simulink model "modelo_1"  (R2023a)
settings: Solver=ode45  StartTime=0.0  StopTime=100  RelTol=1e-3
InitFcn:
  | clc;clear;close all;
  | parametros;
  | FC_detectores;
  | gen_suelo;
  | gain_CL;
values from neighbouring files (symbols this model uses):
  b_cx = 1e6    (= 1000000)    [parametros.m]
  b_cy = 1e7    (= 10000000)    [parametros.m]
  b_ha = (n_h*w_des_h+2*dseta_h*w_des_h)*(J_hEq)-b_hEq    [gain_CL.m]
  b_hb = 1e8    (= 100000000)    [parametros.m]
  b_hd = 8    [parametros.m]
  b_hEb = 2.2e9    (= 2200000000)    [parametros.m]
  b_hm = 18    [parametros.m]
  b_t = 90    [parametros.m]
  b_ta = (n_t*w_des_t+2*dseta_t*w_des_t)*(J_tEq)-b_tEq    [gain_CL.m]
  b_tb = 5e6    (= 5000000)    [parametros.m]
  b_td = 1.8    [parametros.m]
  b_tEq = b_tm+(b_td/i_t^2)+(b_t*r_td^2/i_t^2)    (= 6.027)    [parametros.m]
  b_tm = 6    [parametros.m]
  b_tw = 3e3    (= 3000)    [parametros.m]
  b_wu = 150    [parametros.m]
  FC_e = 1    [FC_detectores.m]
  g = 9.80664    [parametros.m]
  H_c = 2.5    [parametros.m]
  i_h = 22    [parametros.m]
  i_t = 30    [parametros.m]
  J_hd_hEb = 3800    [parametros.m]
  J_hm_hb = 30    [parametros.m]
  J_td = 1200    [parametros.m]
  J_tEq = J_tm_tb+(J_td/i_t^2)+((M_t)*r_td^2/i_t^2)+m_l*r_td^2/i_t^2    (= 20.8333333333)    [parametros.m]
  J_tm_tb = 7    [parametros.m]
  K_cy = 1.8e9    (= 1800000000)    [parametros.m]
  k_hsa = (w_des_h^2+2*dseta_h*w_des_h)*(J_hEq)    [gain_CL.m]
  k_hsia = (w_des_h^3)*(J_hEq)    [gain_CL.m]
  k_tsa = (w_des_t^2+2*dseta_t*w_des_t)*(J_tEq)    [gain_CL.m]
  k_tsia = (w_des_t^3)*(J_tEq)    [gain_CL.m]
  K_tw = 4.8e5    (= 480000)    [parametros.m]
  k_wu = 2.35e8    (= 235000000)    [parametros.m]
  M_cmax = 50000    [parametros.m]
  M_cmin = 2000    [parametros.m]
  M_s = 15000    [parametros.m]
  M_t = 30000    [parametros.m]
  r_hd = 0.75    [parametros.m]
  r_td = 0.50    (= 0.5)    [parametros.m]
  res = 0.01    [gen_suelo.m]
  T_hEbMax = 1.1e6    (= 1100000)    [parametros.m]
  T_s = (b_hEq/J_hEq)/2/pi/100    (= 0.000679331161018)    [parametros.m]
  T_tbMax = 5e3    (= 5000)    [parametros.m]
  v_hMax_loaded = 1.5    [FC_detectores.m]
  v_hMax_over = 1.15    [FC_detectores.m]
  v_hMax_unloaded = 3    [FC_detectores.m]
  x_tMax = 50    [FC_detectores.m]
  x_tMin = -30    [FC_detectores.m]
  y_hMax = 40    [FC_detectores.m]
  y_hMin = -20    [FC_detectores.m]
  Y_t0 = 45    [parametros.m]
libraries: simulink x10
settings Model: Creator=Usuario  LastModifiedBy=Usuario

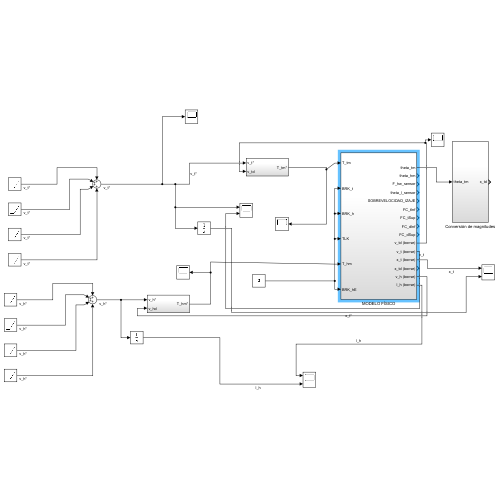
[thumbnail: Simulink's stored preview of the top-level diagram]
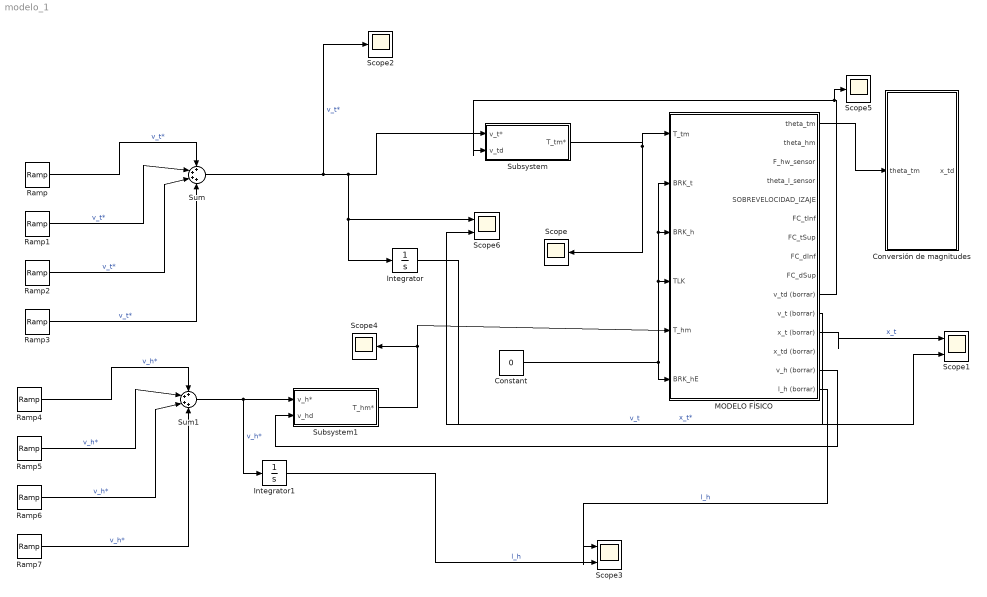
== system modelo_1 ==
  Constant : Constant  Value=0
  Conversión de magnitudes : Subsystem
  Integrator : Integrator
  Integrator1 : Integrator
  MODELO FÍSICO : Subsystem
  Ramp : simulink/Sources/Ramp  slope=0.8  start=5  InitialOutput=0
  Ramp1 : simulink/Sources/Ramp  slope=-0.8  start=10  InitialOutput=0
  Ramp2 : simulink/Sources/Ramp  slope=-0.8  start=35  InitialOutput=0
  Ramp3 : simulink/Sources/Ramp  slope=0.8  start=40  InitialOutput=0
  Ramp4 : simulink/Sources/Ramp  slope=0.8  start=0  InitialOutput=0
  Ramp5 : simulink/Sources/Ramp  slope=-0.8  start=5  InitialOutput=0
  Ramp6 : simulink/Sources/Ramp  slope=-0.8  start=30  InitialOutput=0
  Ramp7 : simulink/Sources/Ramp  slope=0.8  start=35  InitialOutput=0
  Scope{,2,4..5} (4 alike) : Scope
  Scope1 : Scope  NumInputPorts=2
  Scope3 : Scope  NumInputPorts=2
  Scope6 : Scope  NumInputPorts=2
  Subsystem : Subsystem
  Subsystem1 : Subsystem
  Sum : Sum  Inputs=++++
  Sum1 : Sum  Inputs=++++
  wires:
  Constant/1 -> MODELO FÍSICO/6(BRK_hE), MODELO FÍSICO/2(BRK_t), MODELO FÍSICO/3(BRK_h), MODELO FÍSICO/4(TLK)
  Subsystem/1(T_tm*) -> Scope/1, MODELO FÍSICO/1(T_tm)
  MODELO FÍSICO/1(theta_tm) -> Conversión de magnitudes/1(theta_tm)
  MODELO FÍSICO/12(x_t (borrar)) -> Scope1/1  "x_t"
  Sum/1 -> Integrator/1, Scope6/1, Subsystem/1(v_t*), Scope2/1  "v_t*"
  Ramp/1 -> Sum/1  "v_t*"
  Ramp1/1 -> Sum/2  "v_t*"
  Ramp2/1 -> Sum/3  "v_t*"
  Ramp3/1 -> Sum/4  "v_t*"
  MODELO FÍSICO/10(v_td (borrar)) -> Scope5/1, Subsystem/2(v_td)
  Integrator/1 -> Scope1/2  "x_t*"
  Ramp7/1 -> Sum1/4  "v_h*"
  Ramp5/1 -> Sum1/2  "v_h*"
  Ramp4/1 -> Sum1/1  "v_h*"
  Ramp6/1 -> Sum1/3  "v_h*"
  Sum1/1 -> Integrator1/1, Subsystem1/1(v_h*)  "v_h*"
  MODELO FÍSICO/14(v_h (borrar)) -> Subsystem1/2(v_hd)
  Subsystem1/1(T_hm*) -> Scope4/1, MODELO FÍSICO/5(T_hm)
  MODELO FÍSICO/15(l_h (borrar)) -> Scope3/1  "l_h"
  Integrator1/1 -> Scope3/2  "l_h"
  MODELO FÍSICO/11(v_t (borrar)) -> Scope6/2  "v_t"

== system modelo_1/Conversión de magnitudes ==
  theta_tm : Inport
  Gain : Gain  Gain=r_td/i_t
  x_td : Outport
  wires:
  theta_tm/1 -> Gain/1
  Gain/1 -> x_td/1

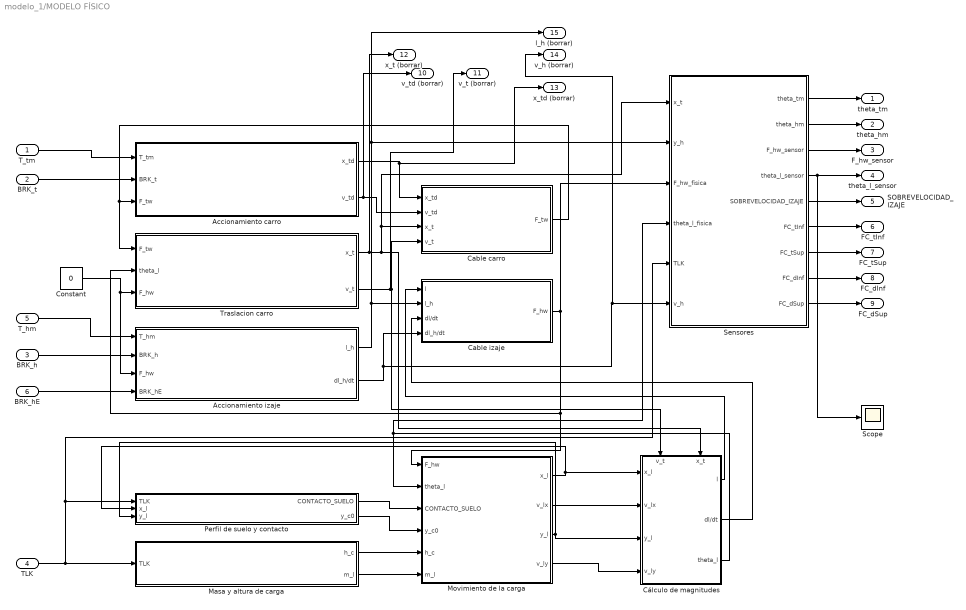
== system modelo_1/MODELO FÍSICO ==
  T_tm : Inport
  BRK_t : Inport  Port=2
  BRK_h : Inport  Port=3
  TLK : Inport  Port=4
  T_hm : Inport  Port=5
  BRK_hE : Inport  Port=6
  Accionamiento carro : Subsystem
  Accionamiento izaje : Subsystem
  Cable carro : Subsystem
  Cable izaje : Subsystem
  Constant : Constant  Value=0
  Cálculo de magnitudes : Subsystem
      settings: PortSchema="{\"entries\":[{\"content\":{\"sides\":[{\"content\":{\"connectorIds\":[\"In1\",\"In2\",\"In3\",\"In4\"]},\"type\":\"ConnectorPlacement.EquallySpacedRectSide\",\"uuid\":\"493eab02-1936-4cf9-830d-aa839ab91fc4\"},{\"content\":{\"connectorIds\":[\"Out1\",\"Out2\",\"Out3\"],\"side\":\"RIGHT\"},\"type\":\"ConnectorPlacement.EquallySpacedRectSide\",\"uuid\":\"61a8ab5c-988b-4ae1-aa5a-5d4cc1e8114e\"},{\"content\":{\"connectorIds\":[\"In5\",\"In6\"],\"side\":\"TOP\"},\"type\":\"ConnectorPlacement.EquallySpacedRectSide\",\"uuid\":\"7fd4977c-3bce-4f08-aaf8-7248d4aa69d5\"}]},\"type\":\"ConnectorPlacement.EquallySpacedConnector\",\"uuid\":\"0caff8b2-9bf4-4a5a-b33d-8eed0c6aecd7\"}],\"packageUris\":[\"http://schema.mathworks.com/mf0/Connector/R2020b\"],\"version\":\"1.0\"}"
  Masa y altura de carga : Subsystem
  Movimiento de la carga : Subsystem
  Perfil de suelo y contacto : Subsystem
  Scope : Scope
  Sensores : Subsystem
  Traslacion carro : Subsystem
  theta_tm : Outport
  theta_hm : Outport  Port=2
  F_hw_sensor : Outport  Port=3
  theta_l_sensor : Outport  Port=4
  SOBREVELOCIDAD_IZAJE : Outport  Port=5
  FC_tInf : Outport  Port=6
  FC_tSup : Outport  Port=7
  FC_dInf : Outport  Port=8
  FC_dSup : Outport  Port=9
  v_td (borrar) : Outport  Port=10
  v_t (borrar) : Outport  Port=11
  x_t (borrar) : Outport  Port=12
  x_td (borrar) : Outport  Port=13
  v_h (borrar) : Outport  Port=14
  l_h (borrar) : Outport  Port=15
  wires:
  TLK/1 -> Sensores/5(TLK), Perfil de suelo y contacto/1(TLK), Masa y altura de carga/1(TLK)
  Accionamiento izaje/1(l_h) -> l_h (borrar)/1, Sensores/2(y_h), Cable izaje/2(l_h)
  Cálculo de magnitudes/3(theta_l) -> Movimiento de la carga/2(theta_l), Sensores/4(theta_l_fisica)
  Accionamiento izaje/2(dl_h/dt) -> Cable izaje/4(dl_h/dt), v_h (borrar)/1, Sensores/6(v_h)
  T_tm/1 -> Accionamiento carro/1(T_tm)
  Sensores/9(FC_dSup) -> FC_dSup/1
  Sensores/2(theta_hm) -> theta_hm/1
  Accionamiento carro/2(v_td) -> v_td (borrar)/1, Cable carro/2(v_td)
  Cálculo de magnitudes/1(l) -> Cable izaje/1(l)
  Perfil de suelo y contacto/2(y_c0) -> Movimiento de la carga/4(y_c0)
  Cable carro/1(F_tw) -> Traslacion carro/1(F_tw), Accionamiento carro/3(F_tw)
  BRK_t/1 -> Accionamiento carro/2(BRK_t)
  Sensores/5(SOBREVELOCIDAD_IZAJE) -> SOBREVELOCIDAD_IZAJE/1
  Sensores/7(FC_tSup) -> FC_tSup/1
  Sensores/1(theta_tm) -> theta_tm/1
  Traslacion carro/1(x_t) -> x_t (borrar)/1, Cálculo de magnitudes/6(x_t), Sensores/1(x_t), Cable carro/3(x_t)
  Cálculo de magnitudes/2(dl/dt) -> Cable izaje/3(dl/dt)
  Sensores/3(F_hw_sensor) -> F_hw_sensor/1
  Sensores/6(FC_tInf) -> FC_tInf/1
  Perfil de suelo y contacto/1(CONTACTO_SUELO) -> Movimiento de la carga/3(CONTACTO_SUELO)
  Movimiento de la carga/2(v_lx) -> Cálculo de magnitudes/2(v_lx)
  Movimiento de la carga/4(v_ly) -> Cálculo de magnitudes/4(v_ly)
  Sensores/8(FC_dInf) -> FC_dInf/1
  Traslacion carro/2(v_t) -> v_t (borrar)/1, Cálculo de magnitudes/5(v_t), Cable carro/4(v_t)
  Accionamiento carro/1(x_td) -> x_td (borrar)/1, Cable carro/1(x_td)
  BRK_h/1 -> Accionamiento izaje/2(BRK_h)
  Movimiento de la carga/3(y_l) -> Perfil de suelo y contacto/3(y_l), Cálculo de magnitudes/3(y_l)
  T_hm/1 -> Accionamiento izaje/1(T_hm)
  Sensores/4(theta_l_sensor) -> theta_l_sensor/1, Scope/1
  BRK_hE/1 -> Accionamiento izaje/4(BRK_hE)
  Masa y altura de carga/1(h_c) -> Movimiento de la carga/5(h_c)
  Movimiento de la carga/1(x_l) -> Perfil de suelo y contacto/2(x_l), Cálculo de magnitudes/1(x_l)
  Masa y altura de carga/2(m_l) -> Movimiento de la carga/6(m_l)
  Cable izaje/1(F_hw) -> Traslacion carro/2(theta_l), Movimiento de la carga/1(F_hw), Sensores/3(F_hw_fisica)
  Constant/1 -> Accionamiento izaje/3(F_hw), Traslacion carro/3(F_hw)

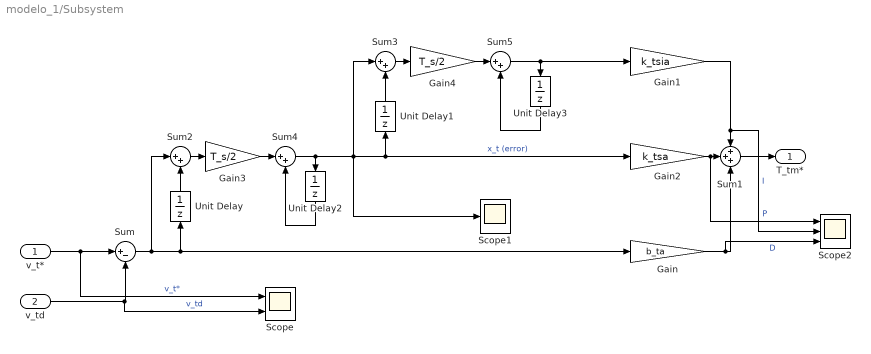
== system modelo_1/Subsystem ==
  v_t* : Inport
  v_td : Inport  Port=2
  Gain : Gain  Gain=b_ta
  Gain1 : Gain  Gain=k_tsia
  Gain2 : Gain  Gain=k_tsa
  Gain3 : Gain  Gain=T_s/2
  Gain4 : Gain  Gain=T_s/2
  Scope : Scope  NumInputPorts=2
  Scope1 : Scope
  Scope2 : Scope  NumInputPorts=3
  Sum : Sum  Inputs=|+-
  Sum1 : Sum  Inputs=+++
  Sum{2..5} (4 alike) : Sum  Inputs=|++
  Unit Delay{,1..3} (4 alike) : UnitDelay  SampleTime=-1  HasFrameUpgradeWarning=on
  T_tm* : Outport
  wires:
  v_t*/1 -> Scope/1, Sum/1  "v_t*"
  v_td/1 -> Scope/2, Sum/2  "v_td"
  Sum/1 -> Sum2/1, Unit Delay/1, Gain/1
  Gain/1 -> Scope2/3, Sum1/3  "D"
  Gain2/1 -> Scope2/1, Sum1/2  "P"
  Gain1/1 -> Scope2/2, Sum1/1  "I"
  Sum1/1 -> T_tm*/1
  Unit Delay1/1 -> Sum3/2
  Unit Delay/1 -> Sum2/2
  Sum2/1 -> Gain3/1
  Sum3/1 -> Gain4/1
  Gain4/1 -> Sum5/1
  Sum4/1 -> Unit Delay2/1, Sum3/1, Scope1/1, Gain2/1, Unit Delay1/1  "x_t (error)"
  Gain3/1 -> Sum4/1
  Unit Delay2/1 -> Sum4/2
  Sum5/1 -> Gain1/1, Unit Delay3/1
  Unit Delay3/1 -> Sum5/2

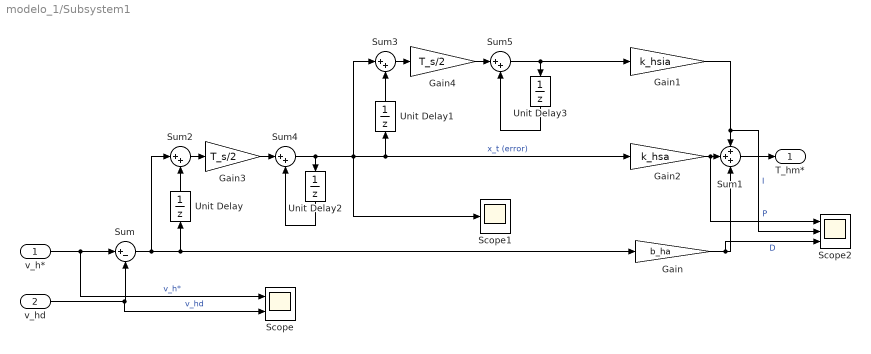
== system modelo_1/Subsystem1 ==
  v_h* : Inport
  v_hd : Inport  Port=2
  Gain : Gain  Gain=b_ha
  Gain1 : Gain  Gain=k_hsia
  Gain2 : Gain  Gain=k_hsa
  Gain3 : Gain  Gain=T_s/2
  Gain4 : Gain  Gain=T_s/2
  Scope : Scope  NumInputPorts=2
  Scope1 : Scope
  Scope2 : Scope  NumInputPorts=3
  Sum : Sum  Inputs=|+-
  Sum1 : Sum  Inputs=+++
  Sum{2..5} (4 alike) : Sum  Inputs=|++
  Unit Delay{,1..3} (4 alike) : UnitDelay  SampleTime=-1  HasFrameUpgradeWarning=on
  T_hm* : Outport
  wires:
  v_h*/1 -> Scope/1, Sum/1  "v_h*"
  v_hd/1 -> Scope/2, Sum/2  "v_hd"
  Sum/1 -> Sum2/1, Unit Delay/1, Gain/1
  Gain/1 -> Scope2/3, Sum1/3  "D"
  Gain2/1 -> Scope2/1, Sum1/2  "P"
  Gain1/1 -> Scope2/2, Sum1/1  "I"
  Sum1/1 -> T_hm*/1
  Unit Delay1/1 -> Sum3/2
  Unit Delay/1 -> Sum2/2
  Sum2/1 -> Gain3/1
  Sum3/1 -> Gain4/1
  Gain4/1 -> Sum5/1
  Sum4/1 -> Unit Delay2/1, Sum3/1, Scope1/1, Gain2/1, Unit Delay1/1  "x_t (error)"
  Gain3/1 -> Sum4/1
  Unit Delay2/1 -> Sum4/2
  Sum5/1 -> Gain1/1, Unit Delay3/1
  Unit Delay3/1 -> Sum5/2

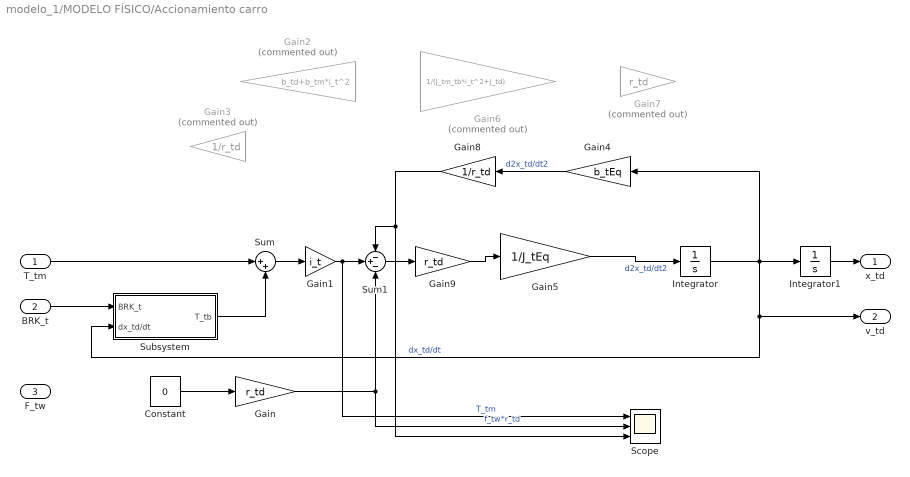
== system modelo_1/MODELO FÍSICO/Accionamiento carro ==
  T_tm : Inport
  BRK_t : Inport  Port=2
  F_tw : Inport  Port=3
  Constant : Constant  Value=0
  Gain : Gain  Gain=r_td
  Gain1 : Gain  Gain=i_t
  Gain2 : Gain  Commented=on  Gain=b_td+b_tm*i_t^2
  Gain3 : Gain  Commented=on  Gain=1/r_td
  Gain4 : Gain  Gain=b_tEq
  Gain5 : Gain  Gain=1/J_tEq
  Gain6 : Gain  Commented=on  Gain=1/(J_tm_tb*i_t^2+J_td)
  Gain7 : Gain  Commented=on  Gain=r_td
  Gain8 : Gain  Gain=1/r_td
  Gain9 : Gain  Gain=r_td
  Integrator : Integrator
  Integrator1 : Integrator
  Scope : Scope  NumInputPorts=3
  Subsystem : Subsystem
  Sum : Sum  Inputs=|++
  Sum1 : Sum  Inputs=-+-
  x_td : Outport
  v_td : Outport  Port=2
  wires:
  T_tm/1 -> Sum/1
  Sum/1 -> Gain1/1
  Gain1/1 -> Scope/1, Sum1/2  "T_tm"
  Gain/1 -> Sum1/3, Scope/2  "f_tw*r_td"
  Integrator/1 -> Gain4/1, Integrator1/1, v_td/1, Subsystem/2(dx_td/dt)  "dx_td/dt"
  Sum1/1 -> Gain9/1
  Gain5/1 -> Integrator/1  "d2x_td/dt2"
  BRK_t/1 -> Subsystem/1(BRK_t)
  Subsystem/1(T_tb) -> Sum/2
  Integrator1/1 -> x_td/1
  Constant/1 -> Gain/1
  Gain4/1 -> Gain8/1  "d2x_td/dt2"
  Gain9/1 -> Gain5/1
  Gain8/1 -> Sum1/1, Scope/3

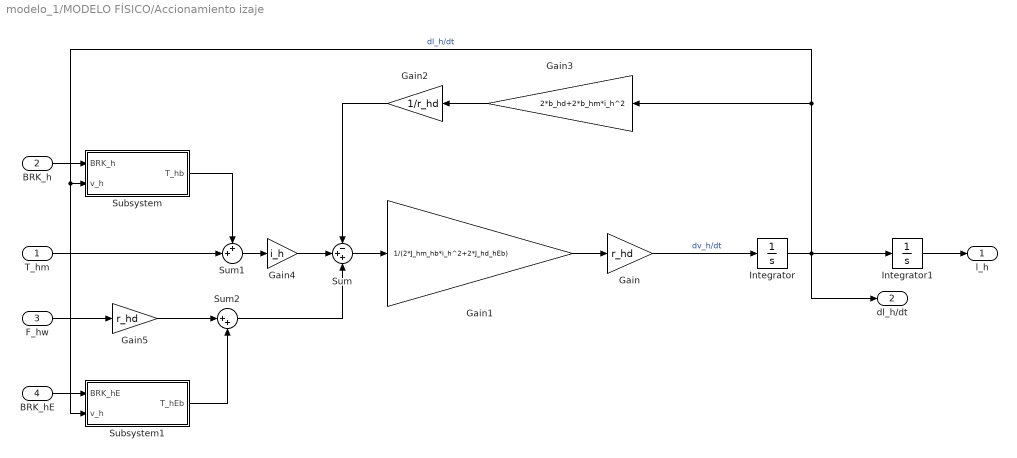
== system modelo_1/MODELO FÍSICO/Accionamiento izaje ==
  T_hm : Inport
  BRK_h : Inport  Port=2
  F_hw : Inport  Port=3
  BRK_hE : Inport  Port=4
  Gain : Gain  Gain=r_hd
  Gain1 : Gain  Gain=1/(2*J_hm_hb*i_h^2+2*J_hd_hEb)
  Gain2 : Gain  Gain=1/r_hd
  Gain3 : Gain  Gain=2*b_hd+2*b_hm*i_h^2
  Gain4 : Gain  Gain=i_h
  Gain5 : Gain  Gain=r_hd
  Integrator : Integrator
  Integrator1 : Integrator
  Subsystem : Subsystem
  Subsystem1 : Subsystem
  Sum : Sum  Inputs=-++
  Sum1 : Sum  Inputs=++|
  Sum2 : Sum  Inputs=|++
  l_h : Outport
  dl_h/dt : Outport  Port=2
  wires:
  Gain/1 -> Integrator/1  "dv_h/dt"
  Gain1/1 -> Gain/1
  Gain3/1 -> Gain2/1
  Integrator/1 -> dl_h/dt/1, Integrator1/1, Gain3/1, Subsystem/2(v_h), Subsystem1/2(v_h)  "dl_h/dt"
  Sum/1 -> Gain1/1
  Gain2/1 -> Sum/1
  Gain4/1 -> Sum/2
  BRK_h/1 -> Subsystem/1(BRK_h)
  Sum1/1 -> Gain4/1
  Subsystem/1(T_hb) -> Sum1/1
  T_hm/1 -> Sum1/2
  F_hw/1 -> Gain5/1
  Gain5/1 -> Sum2/1
  BRK_hE/1 -> Subsystem1/1(BRK_hE)
  Subsystem1/1(T_hEb) -> Sum2/2
  Sum2/1 -> Sum/3
  Integrator1/1 -> l_h/1

== system modelo_1/MODELO FÍSICO/Cable carro ==
  x_td : Inport
  v_td : Inport  Port=2
  x_t : Inport  Port=3
  v_t : Inport  Port=4
  Gain : Gain  Gain=b_tw
  Gain1 : Gain  Gain=K_tw
  Sum : Sum  Inputs=|+-
  Sum1 : Sum  Inputs=|+-
  Sum2 : Sum  Inputs=|++
  F_tw : Outport
  wires:
  Sum/1 -> Gain1/1
  x_td/1 -> Sum/1
  x_t/1 -> Sum/2
  Sum1/1 -> Gain/1
  v_td/1 -> Sum1/1
  v_t/1 -> Sum1/2
  Gain/1 -> Sum2/2
  Gain1/1 -> Sum2/1
  Sum2/1 -> F_tw/1

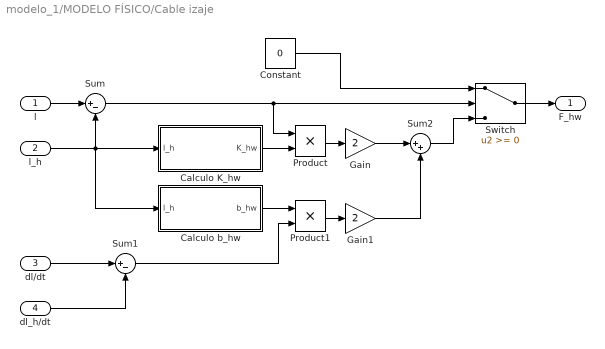
== system modelo_1/MODELO FÍSICO/Cable izaje ==
  l : Inport
  l_h : Inport  Port=2
  dl/dt : Inport  Port=3
  dl_h/dt : Inport  Port=4
  Calculo K_hw : Subsystem
  Calculo b_hw : Subsystem
  Constant : Constant  Value=0
  Gain : Gain  Gain=2
  Gain1 : Gain  Gain=2
  Product : Product
  Product1 : Product
  Sum : Sum  Inputs=|+-
  Sum1 : Sum  Inputs=|+-
  Sum2 : Sum  Inputs=|++
  Switch : Switch  SaturateOnIntegerOverflow=off  InputSameDT=off
  F_hw : Outport
  wires:
  l/1 -> Sum/1
  l_h/1 -> Calculo b_hw/1(l_h), Calculo K_hw/1(l_h), Sum/2
  Sum/1 -> Product/1, Switch/2
  Constant/1 -> Switch/1
  Calculo K_hw/1(K_hw) -> Product/2
  Product/1 -> Gain/1
  dl_h/dt/1 -> Sum1/2
  dl/dt/1 -> Sum1/1
  Product1/1 -> Gain1/1
  Calculo b_hw/1(b_hw) -> Product1/1
  Sum1/1 -> Product1/2
  Gain1/1 -> Sum2/2
  Gain/1 -> Sum2/1
  Sum2/1 -> Switch/3
  Switch/1 -> F_hw/1

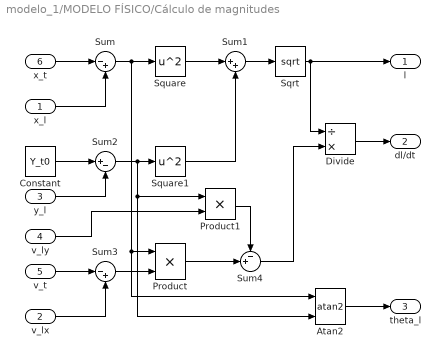
== system modelo_1/MODELO FÍSICO/Cálculo de magnitudes ==
  x_l : Inport
  v_lx : Inport  Port=2
  y_l : Inport  Port=3
  v_ly : Inport  Port=4
  v_t : Inport  Port=5
  x_t : Inport  Port=6
  Atan2 : Trigonometry  Operator=atan2
  Constant : Constant  Value=Y_t0
  Divide : Product  Inputs=/*
  Product : Product
  Product1 : Product
  Sqrt : Sqrt
  Square : Math  Operator=square
  Square1 : Math  Operator=square
  Sum : Sum  Inputs=|-+
  Sum1 : Sum  Inputs=|++
  Sum2 : Sum  Inputs=|+-
  Sum3 : Sum  Inputs=|-+
  Sum4 : Sum  Inputs=-+|
  l : Outport
  dl/dt : Outport  Port=2
  theta_l : Outport  Port=3
  wires:
  x_t/1 -> Sum/1
  x_l/1 -> Sum/2
  Square/1 -> Sum1/1
  Constant/1 -> Sum2/1
  y_l/1 -> Sum2/2
  Sum2/1 -> Atan2/2, Product1/1, Square1/1
  Square1/1 -> Sum1/2
  Sum1/1 -> Sqrt/1
  Sqrt/1 -> Divide/1, l/1
  v_t/1 -> Sum3/1
  v_lx/1 -> Sum3/2
  Sum3/1 -> Product/2
  Product/1 -> Sum4/2
  v_ly/1 -> Product1/2
  Product1/1 -> Sum4/1
  Sum4/1 -> Divide/2
  Divide/1 -> dl/dt/1
  Atan2/1 -> theta_l/1
  Sum/1 -> Product/1, Atan2/1, Square/1

== system modelo_1/MODELO FÍSICO/Masa y altura de carga ==
  TLK : Inport
  Constant : Constant  Value=0
  Constant1 : Constant  Value=H_c
  Constant2 : Constant  Value=M_s
  M_cx : UniformRandomNumber  Minimum=M_cmin  Maximum=M_cmax  SampleTime=0.1
  Sum : Sum  Inputs=|++
  Switch : Switch  Criteria=u2 > Threshold  SaturateOnIntegerOverflow=off  InputSameDT=off
  Switch1 : Switch  Criteria=u2 > Threshold  SaturateOnIntegerOverflow=off  InputSameDT=off
  h_c : Outport
  m_l : Outport  Port=2
  wires:
  TLK/1 -> Switch/2, Switch1/2
  Constant/1 -> Switch/1
  Switch/1 -> h_c/1
  Constant1/1 -> Switch/3
  Switch1/1 -> m_l/1
  Constant2/1 -> Switch1/3, Sum/1
  M_cx/1 -> Sum/2
  Sum/1 -> Switch1/1

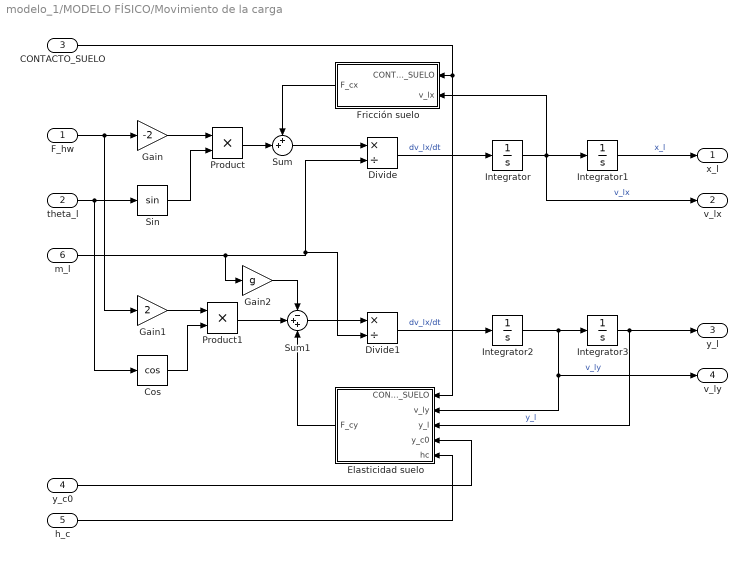
== system modelo_1/MODELO FÍSICO/Movimiento de la carga ==
  F_hw : Inport
  theta_l : Inport  Port=2
  CONTACTO_SUELO : Inport  Port=3
  y_c0 : Inport  Port=4
  h_c : Inport  Port=5
  m_l : Inport  Port=6
  Cos : Trigonometry  Operator=cos
  Divide : Product  Inputs=*/
  Divide1 : Product  Inputs=*/
  Elasticidad suelo : Subsystem
  Fricción suelo : Subsystem
  Gain : Gain  Gain=-2
  Gain1 : Gain  Gain=2
  Gain2 : Gain  Gain=g
  Integrator{,1..3} (4 alike) : Integrator
  Product : Product
  Product1 : Product
  Sin : Trigonometry
  Sum : Sum  Inputs=++|
  Sum1 : Sum  Inputs=-++
  x_l : Outport
  v_lx : Outport  Port=2
  y_l : Outport  Port=3
  v_ly : Outport  Port=4
  wires:
  F_hw/1 -> Gain1/1, Gain/1
  Gain/1 -> Product/1
  theta_l/1 -> Cos/1, Sin/1
  Sin/1 -> Product/2
  Product/1 -> Sum/2
  Divide/1 -> Integrator/1  "dv_lx/dt"
  Fricción suelo/1(F_cx) -> Sum/1
  Integrator/1 -> v_lx/1, Integrator1/1, Fricción suelo/2(v_lx)  "v_lx"
  CONTACTO_SUELO/1 -> Elasticidad suelo/1(CONTACTO_SUELO), Fricción suelo/1(CONTACTO_SUELO)
  Sum/1 -> Divide/1
  m_l/1 -> Gain2/1, Divide1/2, Divide/2
  Integrator1/1 -> x_l/1  "x_l"
  Gain1/1 -> Product1/1
  Cos/1 -> Product1/2
  Product1/1 -> Sum1/2
  Elasticidad suelo/1(F_cy) -> Sum1/3
  Integrator3/1 -> Elasticidad suelo/3(y_l), y_l/1  "y_l"
  Integrator2/1 -> Elasticidad suelo/2(v_ly), v_ly/1, Integrator3/1  "v_ly"
  Sum1/1 -> Divide1/1
  Divide1/1 -> Integrator2/1  "dv_lx/dt"
  Gain2/1 -> Sum1/1
  h_c/1 -> Elasticidad suelo/5(hc)
  y_c0/1 -> Elasticidad suelo/4(y_c0)

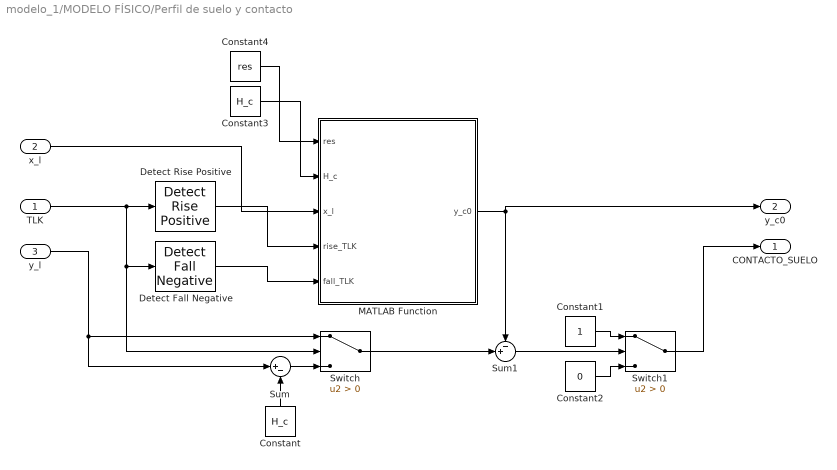
== system modelo_1/MODELO FÍSICO/Perfil de suelo y contacto ==
  TLK : Inport
  x_l : Inport  Port=2
  y_l : Inport  Port=3
  Constant : Constant  Value=H_c
  Constant1 : Constant
  Constant2 : Constant  Value=0
  Constant3 : Constant  Value=H_c
  Constant4 : Constant  Value=res
  Detect Fall Negative : simulink/Logic and Bit Operations/Detect Fall Negative  vinit=0  OutDataTypeStr=boolean
  Detect Rise Positive : simulink/Logic and Bit Operations/Detect Rise Positive  vinit=0  OutDataTypeStr=boolean
  MATLAB Function : MATLAB Function  TreatAsAtomicUnit=on
  Sum : Sum  Inputs=|+-
  Sum1 : Sum  Inputs=-+|
  Switch : Switch  Criteria=u2 > Threshold  SaturateOnIntegerOverflow=off  InputSameDT=off
  Switch1 : Switch  Criteria=u2 > Threshold  SaturateOnIntegerOverflow=off  InputSameDT=off
  CONTACTO_SUELO : Outport
  y_c0 : Outport  Port=2
  wires:
  TLK/1 -> Switch/2, Detect Fall Negative/1, Detect Rise Positive/1
  Detect Rise Positive/1 -> MATLAB Function/4(rise_TLK)
  Detect Fall Negative/1 -> MATLAB Function/5(fall_TLK)
  x_l/1 -> MATLAB Function/3(x_l)
  MATLAB Function/1(y_c0) -> y_c0/1, Sum1/1
  y_l/1 -> Sum/1, Switch/1
  Sum/1 -> Switch/3
  Constant/1 -> Sum/2
  Switch/1 -> Sum1/2
  Sum1/1 -> Switch1/2
  Constant1/1 -> Switch1/1
  Constant2/1 -> Switch1/3
  Switch1/1 -> CONTACTO_SUELO/1
  Constant3/1 -> MATLAB Function/2(H_c)
  Constant4/1 -> MATLAB Function/1(res)

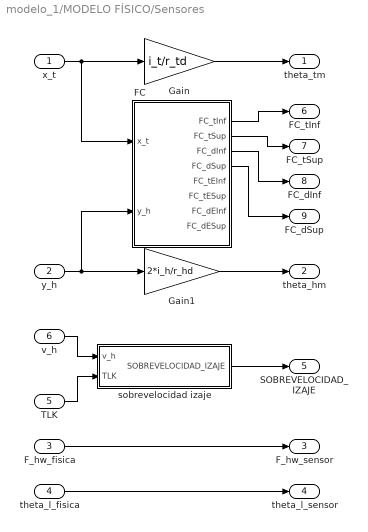
== system modelo_1/MODELO FÍSICO/Sensores ==
  x_t : Inport
  y_h : Inport  Port=2
  F_hw_fisica : Inport  Port=3
  theta_l_fisica : Inport  Port=4
  TLK : Inport  Port=5
  v_h : Inport  Port=6
  FC : Subsystem
  Gain : Gain  Gain=i_t/r_td
  Gain1 : Gain  Gain=2*i_h/r_hd
  sobrevelocidad izaje : Subsystem
  theta_tm : Outport
  theta_hm : Outport  Port=2
  F_hw_sensor : Outport  Port=3
  theta_l_sensor : Outport  Port=4
  SOBREVELOCIDAD_IZAJE : Outport  Port=5
  FC_tInf : Outport  Port=6
  FC_tSup : Outport  Port=7
  FC_dInf : Outport  Port=8
  FC_dSup : Outport  Port=9
  wires:
  x_t/1 -> FC/1(x_t), Gain/1
  Gain/1 -> theta_tm/1
  Gain1/1 -> theta_hm/1
  y_h/1 -> FC/2(y_h), Gain1/1
  F_hw_fisica/1 -> F_hw_sensor/1
  theta_l_fisica/1 -> theta_l_sensor/1
  TLK/1 -> sobrevelocidad izaje/2(TLK)
  sobrevelocidad izaje/1(SOBREVELOCIDAD_IZAJE) -> SOBREVELOCIDAD_IZAJE/1
  v_h/1 -> sobrevelocidad izaje/1(v_h)
  FC/1(FC_tInf) -> FC_tInf/1
  FC/2(FC_tSup) -> FC_tSup/1
  FC/3(FC_dInf) -> FC_dInf/1
  FC/4(FC_dSup) -> FC_dSup/1

== system modelo_1/MODELO FÍSICO/Traslacion carro ==
  F_tw : Inport
  theta_l : Inport  Port=2
  F_hw : Inport  Port=3
  Gain : Gain  Gain=2
  Gain1 : Gain  Gain=b_t
  Gain2 : Gain  Gain=1/M_t
  Integrator : Integrator
  Integrator1 : Integrator
  Product : Product
  Scope : Scope  NumInputPorts=3
  Sin : Trigonometry
  Sum : Sum  Inputs=-++
  x_t : Outport
  v_t : Outport  Port=2
  wires:
  F_tw/1 -> Sum/3, Scope/2
  F_hw/1 -> Gain/1
  Gain/1 -> Product/1
  theta_l/1 -> Sin/1
  Sin/1 -> Product/2
  Product/1 -> Scope/3, Sum/2
  Integrator/1 -> v_t/1, Integrator1/1, Gain1/1  "v_t"
  Sum/1 -> Gain2/1
  Gain2/1 -> Integrator/1  "dv_t/dt"
  Integrator1/1 -> x_t/1
  Gain1/1 -> Scope/1, Sum/1

== system modelo_1/MODELO FÍSICO/Accionamiento carro/Subsystem ==
  BRK_t : Inport
  dx_td/dt : Inport  Port=2
  Constant : Constant  Value=0
  Gain : Gain  Gain=i_t/r_td
  Gain1 : Gain  Gain=b_tb
  Saturation : Saturate  UpperLimit=T_tbMax  LowerLimit=-T_tbMax
  Scope : Scope
  Switch : Switch  Criteria=u2 > Threshold  SaturateOnIntegerOverflow=off  InputSameDT=off
  T_tb : Outport
  wires:
  Saturation/1 -> Scope/1, T_tb/1
  Switch/1 -> Saturation/1
  dx_td/dt/1 -> Gain/1
  Gain/1 -> Gain1/1
  BRK_t/1 -> Switch/2
  Constant/1 -> Switch/3
  Gain1/1 -> Switch/1

== system modelo_1/MODELO FÍSICO/Accionamiento izaje/Subsystem ==
  BRK_h : Inport
  v_h : Inport  Port=2
  Constant : Constant  Value=0
  Gain : Gain  Gain=i_h/r_hd
  Gain1 : Gain  Gain=b_hb
  Saturation : Saturate  UpperLimit=T_hEbMax  LowerLimit=-T_hEbMax
  Switch : Switch  Criteria=u2 > Threshold  SaturateOnIntegerOverflow=off  InputSameDT=off
  T_hb : Outport
  wires:
  BRK_h/1 -> Switch/2
  Switch/1 -> Saturation/1
  Saturation/1 -> T_hb/1
  Constant/1 -> Switch/3
  v_h/1 -> Gain/1
  Gain/1 -> Gain1/1
  Gain1/1 -> Switch/1

== system modelo_1/MODELO FÍSICO/Accionamiento izaje/Subsystem1 ==
  BRK_hE : Inport
  v_h : Inport  Port=2
  Constant : Constant  Value=0
  Gain : Gain  Gain=1/r_hd
  Gain1 : Gain  Gain=b_hEb
  Saturation : Saturate  UpperLimit=T_hEbMax  LowerLimit=-T_hEbMax
  Scope : Scope
  Switch : Switch  Criteria=u2 > Threshold  SaturateOnIntegerOverflow=off  InputSameDT=off
  T_hEb : Outport
  wires:
  BRK_hE/1 -> Switch/2
  Switch/1 -> Scope/1, Saturation/1
  Saturation/1 -> T_hEb/1
  Constant/1 -> Switch/3
  v_h/1 -> Gain/1
  Gain/1 -> Gain1/1
  Gain1/1 -> Switch/1

== system modelo_1/MODELO FÍSICO/Cable izaje/Calculo K_hw ==
  l_h : Inport
  Constant : Constant  Value=110
  Constant1 : Constant  Value=k_wu
  Divide : Product  Inputs=*/
  Gain : Gain  Gain=2
  Sum : Sum  Inputs=|++
  K_hw : Outport
  wires:
  l_h/1 -> Gain/1
  Gain/1 -> Sum/1
  Constant/1 -> Sum/2
  Sum/1 -> Divide/2
  Constant1/1 -> Divide/1
  Divide/1 -> K_hw/1

== system modelo_1/MODELO FÍSICO/Cable izaje/Calculo b_hw ==
  l_h : Inport
  Constant : Constant  Value=110
  Gain : Gain  Gain=2
  Gain1 : Gain  Gain=b_wu
  Sum : Sum  Inputs=|++
  b_hw : Outport
  wires:
  l_h/1 -> Gain/1
  Gain/1 -> Sum/1
  Constant/1 -> Sum/2
  Sum/1 -> Gain1/1
  Gain1/1 -> b_hw/1

== system modelo_1/MODELO FÍSICO/Movimiento de la carga/Elasticidad suelo ==
  CONTACTO_SUELO : Inport
  v_ly : Inport  Port=2
  y_l : Inport  Port=3
  y_c0 : Inport  Port=4
  hc : Inport  Port=5
  Constant : Constant  Value=0
  Gain : Gain  Gain=-b_cy
  Gain1 : Gain  Gain=K_cy
  Sum : Sum  Inputs=|++
  Sum1 : Sum  Inputs=|+-
  Sum2 : Sum  Inputs=-|+
  Switch : Switch  Criteria=u2 > Threshold  SaturateOnIntegerOverflow=off  InputSameDT=off
  F_cy : Outport
  wires:
  v_ly/1 -> Gain/1
  CONTACTO_SUELO/1 -> Switch/2
  Switch/1 -> F_cy/1
  Constant/1 -> Switch/1
  Gain/1 -> Sum/1
  Gain1/1 -> Sum/2
  Sum/1 -> Switch/3
  y_l/1 -> Sum1/1
  hc/1 -> Sum1/2
  Sum1/1 -> Sum2/1
  y_c0/1 -> Sum2/2
  Sum2/1 -> Gain1/1

== system modelo_1/MODELO FÍSICO/Movimiento de la carga/Fricción suelo ==
  CONTACTO_SUELO : Inport
  v_lx : Inport  Port=2
  Constant : Constant  Value=0
  Gain : Gain  Gain=-b_cx
  Switch : Switch  Criteria=u2 > Threshold  SaturateOnIntegerOverflow=off  InputSameDT=off
  F_cx : Outport
  wires:
  v_lx/1 -> Gain/1
  CONTACTO_SUELO/1 -> Switch/2
  Switch/1 -> F_cx/1
  Gain/1 -> Switch/3
  Constant/1 -> Switch/1

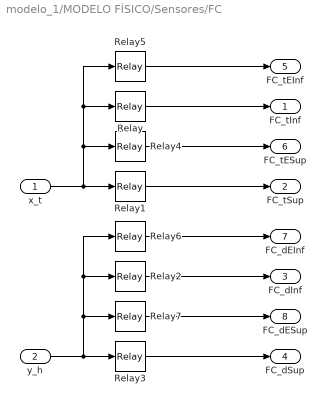
== system modelo_1/MODELO FÍSICO/Sensores/FC ==
  x_t : Inport
  y_h : Inport  Port=2
  Relay : Relay  OnSwitchValue=x_tMin  OffSwitchValue=x_tMin  OnOutputValue=0  OffOutputValue=1
  Relay1 : Relay  OnSwitchValue=x_tMax  OffSwitchValue=x_tMax
  Relay2 : Relay  OnSwitchValue=y_hMin  OffSwitchValue=y_hMin  OnOutputValue=0  OffOutputValue=1
  Relay3 : Relay  OnSwitchValue=y_hMax  OffSwitchValue=y_hMax
  Relay4 : Relay  OnSwitchValue=x_tMax+FC_e  OffSwitchValue=x_tMax+FC_e
  Relay5 : Relay  OnSwitchValue=x_tMin-FC_e  OffSwitchValue=x_tMin-FC_e  OnOutputValue=0  OffOutputValue=1
  Relay6 : Relay  OnSwitchValue=y_hMin-FC_e  OffSwitchValue=y_hMin-FC_e  OnOutputValue=0  OffOutputValue=1
  Relay7 : Relay  OnSwitchValue=y_hMax+FC_e  OffSwitchValue=y_hMax+FC_e
  FC_tInf : Outport
  FC_tSup : Outport  Port=2
  FC_dInf : Outport  Port=3
  FC_dSup : Outport  Port=4
  FC_tEInf : Outport  Port=5
  FC_tESup : Outport  Port=6
  FC_dEInf : Outport  Port=7
  FC_dESup : Outport  Port=8
  wires:
  Relay/1 -> FC_tInf/1
  x_t/1 -> Relay4/1, Relay5/1, Relay/1, Relay1/1
  Relay1/1 -> FC_tSup/1
  Relay3/1 -> FC_dSup/1
  Relay2/1 -> FC_dInf/1
  Relay5/1 -> FC_tEInf/1
  Relay4/1 -> FC_tESup/1
  Relay6/1 -> FC_dEInf/1
  Relay7/1 -> FC_dESup/1
  y_h/1 -> Relay3/1, Relay7/1, Relay6/1, Relay2/1

== system modelo_1/MODELO FÍSICO/Sensores/sobrevelocidad izaje ==
  v_h : Inport
  TLK : Inport  Port=2
  Constant : Constant  Value=v_hMax_loaded
  Constant1 : Constant  Value=v_hMax_unloaded
  Constant2 : Constant  Value=0
  Constant3 : Constant
  Gain : Gain  Gain=v_hMax_over
  Sum : Sum  Inputs=|+-
  Switch : Switch  Criteria=u2 > Threshold  SaturateOnIntegerOverflow=off  InputSameDT=off
  Switch1 : Switch  SaturateOnIntegerOverflow=off  InputSameDT=off
  SOBREVELOCIDAD_IZAJE : Outport
  wires:
  TLK/1 -> Switch/2
  Constant/1 -> Switch/1
  Constant1/1 -> Switch/3
  Switch/1 -> Gain/1
  v_h/1 -> Sum/1
  Gain/1 -> Sum/2
  Sum/1 -> Switch1/2
  Switch1/1 -> SOBREVELOCIDAD_IZAJE/1
  Constant2/1 -> Switch1/3
  Constant3/1 -> Switch1/1

== matlab function modelo_1/MODELO FÍSICO/Perfil de suelo y contacto/MATLAB Function ==
  settings: updateMethod=DISCRETE
  data: res input; H_c input; x_l input; y_c0 output; rise_TLK input; fall_TLK input
function y_c0 = modificar_suelo(res, H_c, x_l, rise_TLK, fall_TLK)
    
    %   rise_TLK  : flag (bool)  -> flanco de subida, tomar carga
    %   fall_TLK  : flag (bool)  -> flanco de bajada, dejar carga
    
    persistent initialized terrain  
    
    if isempty(initialized)
        s        = load('terreno_inicial.mat');   
        terrain  = s.ground_profile;   
        initialized = true;
    end
    
    if rise_TLK || fall_TLK
    
        x_lo = x_l - H_c/2;
        x_hi = x_l + H_c/2;
    
        mask_seg = (terrain(:,1) >=  x_lo - res) & ...
                   (terrain(:,1) <=  x_hi + res);
    
        if rise_TLK
            terrain(mask_seg,2) = terrain(mask_seg,2) + H_c;   
        else  
            terrain(mask_seg,2) = terrain(mask_seg,2) - H_c;   
        end
    end
    
    
    mask = abs(terrain(:,1) - x_l) <= res;
    y_c0 = mean(terrain(mask,2));

end
